simulink model "MPSK_sample_based"  (R2017b)
settings: Solver=FixedStepAuto  StartTime=0.0  StopTime=stopTime  FixedStep=clockTime  RelTol=1e-3
values from neighbouring files (symbols this model uses):
  detectionThreshold = 0.5    [MPSK_frame_based_init.m]    (also in MPSK_sample_based_init.m)
  M = 2^K    (= 4)    [Digital_QAM.m]    (also in MPSK_constellation_decisionRegions.m = 8; MPSK_frame_based_init.m = 2; MPSK_init.m = 2; MPSK_sample_based_init.m = 2)
  phaseOffset = pi    (= 3.14159265359)    [MPSK_frame_based_init.m]    (also in MPSK_init.m = -0.785398163397; MPSK_sample_based_init.m)
  samplesPerSymb = 10    [MPSK_sample_based_init.m]
  sampleTime = 1/sampleRate    (= 0.01)    [MPSK_sample_based_init.m]
undefined symbols (not defined in the file or in its folder): i
libraries: simulink x4, simulink_extras x3, commutil2 x3, dspsigops x2, commfilt2 x2, commchan3 x1, commseqgen3 x1, commsink2 x1, commrflib2 x1
settings Model: Creator=john3  LastModifiedBy=croft

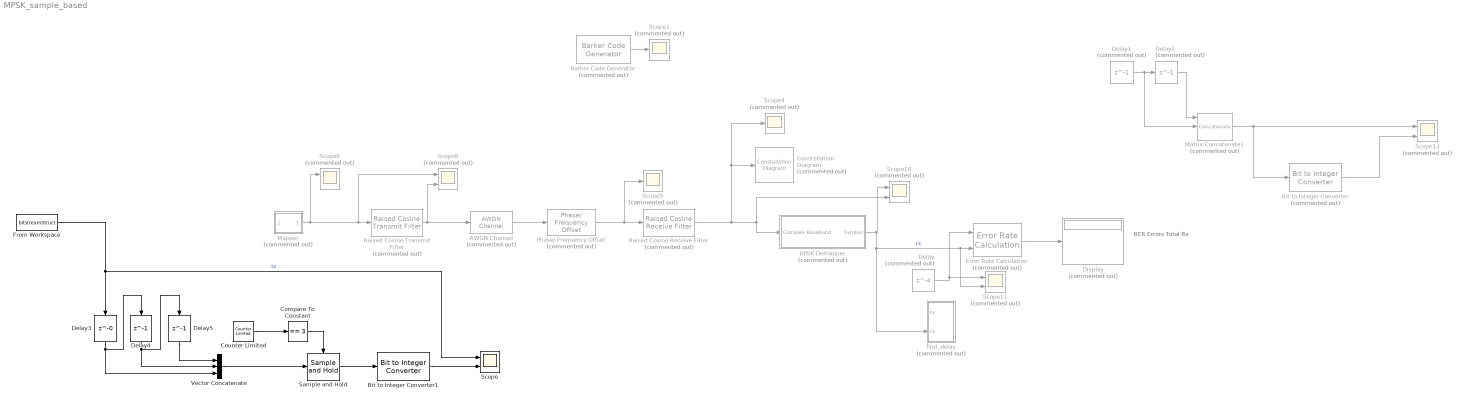
== system MPSK_sample_based ==
  note: BER
      | Errors
      | Total Rx
  AWGN Channel : commchan3/AWGN Channel  Commented=on  InputProcessing=Columns as channels (frame based)  seed=67  noiseMode="Signal to noise ratio  (SNR)"  EbNodB=10  EsNodB=10  SNRdB=30  bitsPerSym=K  Ps=1  Tsym=1  variance=1
  BPSK Demapper : Subsystem  Commented=on
  Barker Code Generator : commseqgen3/Barker Code Generator  Commented=on  Length=7  LengthSimulink=7  SampleTime=1  SamplesPerFrame=1  OutputDataType=double  SimulateUsing=Interpreted execution
      settings: SourceProductName=Communications System Toolbox  SourceProductBaseCode=CM
  Bit to Integer Converter : commutil2/Bit to Integer Converter  Commented=on  nbits=3  bitOrder=MSB first  signedOutputValues=Unsigned  outDtype=Inherit via internal rule  outDtypeSigned=Inherit via internal rule
  Bit to Integer Converter1 : commutil2/Bit to Integer Converter  nbits=3  bitOrder=MSB first  signedOutputValues=Unsigned  outDtype=Inherit via internal rule  outDtypeSigned=Inherit via internal rule
  Compare To Constant : simulink/Logic and Bit Operations/Compare To Constant  relop===  const=3  OutDataTypeStr=boolean
  Constellation Diagram : ConstellationDiagram  Commented=on
  Counter Limited : simulink/Sources/Counter Limited  uplimit=3  tsamp=sampleTime
  Delay : Delay  Commented=on  DelayLength=4
  Delay1 : Delay  Commented=on  DelayLength=1
  Delay2 : Delay  Commented=on  DelayLength=1
  Delay3 : Delay  DelayLength=0
  Delay4 : Delay  DelayLength=1
  Delay5 : Delay  DelayLength=1
  Display : Display  Commented=on
  Error Rate Calculation : commsink2/Error Rate Calculation  Commented=on  N=0  st_delay=0  cp_mode=Entire frame  subframe=[]  PMode=Port  WsName=ErrorVec  RsMode2=off  stop=off  numErr=100  maxBits=1e6
  From Workspace : FromWorkspace  VariableName=bitstreamStruct  SampleTime=sampleTime
  Mapper : Subsystem  Commented=on
  Matrix Concatenate1 : Concatenate  Commented=on  NumInputs=3  ConcatenateDimension=2
  Phase/ Frequency Offset : commrflib2/Phase// Frequency Offset  Commented=on  phaseOffset=phaseOffset*180/pi  freqPort=off  freqOffset=0
      settings: SourceProductName=Communications System Toolbox
  Raised Cosine Receive Filter : commfilt2/Raised Cosine Receive Filter  Commented=on  filtType=Square root  R=1  filtSpan=4  N=samplesPerSymb  downFactor=samplesPerSymb  downOffset=0  filterGain=1  RateOptions=Allow multirate processing  framing=Mute  checkCoeff=off  variableName=rcRxFilt  currentFiltSpan=4  D=(4)/2  inputOffset=0  sampMode=Mute  saveAsFlag=0  rateMode=Downsampling  checkGain=Normalized  launchFVT=on  roundingMode=Floor  overflowMode=off  coeffDataTypeStr=Inherit: Same word length as input  coeffMin=[]  coeffMax=[]  coeffLastDataTypeStr=Inherit: Same word length as input  accumDataTypeStr=Inherit: Same as product output  accumLastDataTypeStr=Inherit: Same as product output  outputDataTypeStr=Inherit: Same as accumulator  outputMin=[]  outputMax=[]  outputLastDataTypeStr=Inherit: Same as accumulator
  Raised Cosine Transmit Filter : commfilt2/Raised Cosine Transmit Filter  Commented=on  filtType=Square root  R=1  filtSpan=4  N=samplesPerSymb  filterGain=1  RateOptions=Allow multirate processing  framing=Mute  checkCoeff=off  variableName=rcTxFilt  checkGain=Normalized  sampMode=Mute  saveAsFlag=0  currentFiltSpan=4  D=(4)/2  launchFVT=on  roundingMode=Floor  overflowMode=off  coeffDataTypeStr=Inherit: Same word length as input  coeffMin=[]  coeffMax=[]  coeffLastDataTypeStr=Inherit: Same word length as input  outputDataTypeStr=Inherit: Same as accumulator  outputMin=[]  outputMax=[]  outputLastDataTypeStr=Inherit: Same as accumulator
  Sample and Hold : dspsigops/Sample and Hold  trig=Rising edge  initCond=0  latchinput=off
  Scope : Scope  NumInputPorts=2
  Scope1 : Scope  Commented=on
  Scope{6,8,10..11,13} (5 alike) : Scope  Commented=on  NumInputPorts=2
  Scope4 : Scope  Commented=on
  Scope9 : Scope  Commented=on
  Vector Concatenate : Concatenate  NumInputs=3
  find_delay : Subsystem  Commented=on
  wires:
  Error Rate Calculation/1 -> Display/1
  Barker Code Generator/1 -> Scope1/1
  AWGN Channel/1 -> Phase/ Frequency Offset/1
  Mapper/1(Out1) -> Scope8/1, Raised Cosine Transmit Filter/1, Scope6/1
  Raised Cosine Transmit Filter/1 -> AWGN Channel/1, Scope8/2
  Phase/ Frequency Offset/1 -> Raised Cosine Receive Filter/1, Scope9/1
  Raised Cosine Receive Filter/1 -> Scope10/2, BPSK Demapper/1(Complex Baseband), Scope4/1, Constellation Diagram/1
  BPSK Demapper/1(Symbol) -> Scope11/2, Error Rate Calculation/2, find_delay/2(rx), Scope10/1  "rx"
  Delay1/1 -> Matrix Concatenate1/2, Delay2/1
  Delay2/1 -> Matrix Concatenate1/1
  Bit to Integer Converter/1 -> Scope13/2
  Matrix Concatenate1/1 -> Scope13/1, Bit to Integer Converter/1
  Delay/1 -> Scope11/1, Error Rate Calculation/1
  From Workspace/1 -> Scope/1, Delay3/1  "tx"
  Delay3/1 -> Vector Concatenate/3, Delay4/1
  Delay4/1 -> Vector Concatenate/2, Delay5/1
  Delay5/1 -> Vector Concatenate/1
  Counter Limited/1 -> Compare To Constant/1
  Compare To Constant/1 -> Sample and Hold/Trigger
  Vector Concatenate/1 -> Sample and Hold/1
  Sample and Hold/1 -> Bit to Integer Converter1/1
  Bit to Integer Converter1/1 -> Scope/2

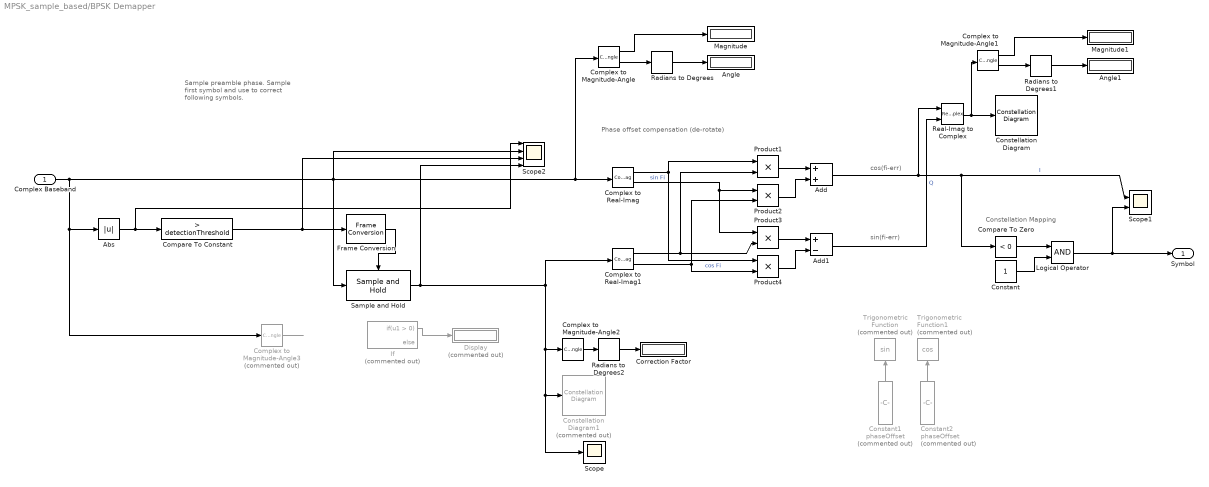
== system MPSK_sample_based/BPSK Demapper ==
  note: cos(fi-err)
  note: Sample preamble phase.
      | Sample first symbol and
      | use to correct following
      | symbols.
  note: Phase offset compensation (de-rotate)
  note: Constellation Mapping
  note: sin(fi-err)
  Complex Baseband : Inport
  Abs : Abs
  Add : Sum
  Add1 : Sum  Inputs=+-
  Angle : Display
  Angle1 : Display
  Compare To Constant : simulink/Logic and Bit Operations/Compare To Constant  relop=>  const=detectionThreshold  OutDataTypeStr=boolean
  Compare To Zero : simulink/Logic and Bit Operations/Compare To Zero  relop=<  OutDataTypeStr=boolean
  Complex to Magnitude-Angle : ComplexToMagnitudeAngle
  Complex to Magnitude-Angle1 : ComplexToMagnitudeAngle
  Complex to Magnitude-Angle2 : ComplexToMagnitudeAngle  Output=Angle
  Complex to Magnitude-Angle3 : ComplexToMagnitudeAngle  Commented=on  Output=Angle
  Complex to Real-Imag : ComplexToRealImag
  Complex to Real-Imag1 : ComplexToRealImag
  Constant : Constant  OutDataTypeStr=boolean
  Constant1 : Constant  Commented=on  Value=phaseOffset
  Constant2 : Constant  Commented=on  Value=phaseOffset
  Constellation Diagram : ConstellationDiagram
  Constellation Diagram1 : ConstellationDiagram  Commented=on
  Correction Factor : Display
  Display : Display  Commented=on
  Frame Conversion : FrameConversion  InheritSamplingMode=off  OutFrame=Sample-based
  If : If  Commented=on
  Logical Operator : Logic  AllPortsSameDT=off  OutDataTypeStr=boolean
  Magnitude : Display
  Magnitude1 : Display
  Product{1..4} (4 alike) : Product
  Radians to Degrees : simulink_extras/Transformations/Radians to Degrees
  Radians to Degrees1 : simulink_extras/Transformations/Radians to Degrees
  Radians to Degrees2 : simulink_extras/Transformations/Radians to Degrees
  Real-Imag to Complex : RealImagToComplex
  Sample and Hold : dspsigops/Sample and Hold  trig=Rising edge  initCond=0  latchinput=off
  Scope : Scope
  Scope1 : Scope  NumInputPorts=2
  Scope2 : Scope  NumInputPorts=4
  Trigonometric Function : Trigonometry  Commented=on
  Trigonometric Function1 : Trigonometry  Commented=on  Operator=cos
  Symbol : Outport
  wires:
  Compare To Zero/1 -> Logical Operator/1
  Complex Baseband/1 -> Sample and Hold/1, Scope2/2, Complex to Magnitude-Angle/1, Complex to Real-Imag/1, Complex to Magnitude-Angle3/1, Abs/1
  Constant/1 -> Logical Operator/2
  Constant1/1 -> Trigonometric Function/1
  Constant2/1 -> Trigonometric Function1/1
  Real-Imag to Complex/1 -> Complex to Magnitude-Angle1/1, Constellation Diagram/1
  Product1/1 -> Add/1
  Product2/1 -> Add/2
  Product3/1 -> Add1/1
  Product4/1 -> Add1/2
  Add/1 -> Compare To Zero/1, Scope1/1, Real-Imag to Complex/1  "I"
  Add1/1 -> Real-Imag to Complex/2  "Q"
  Logical Operator/1 -> Scope1/2, Symbol/1
  Sample and Hold/1 -> Scope2/4, Scope/1, Constellation Diagram1/1, Complex to Magnitude-Angle2/1, Complex to Real-Imag1/1
  Complex to Magnitude-Angle/1 -> Magnitude/1
  Complex to Magnitude-Angle/2 -> Radians to Degrees/1
  Radians to Degrees/1 -> Angle/1
  Radians to Degrees1/1 -> Angle1/1
  Complex to Magnitude-Angle1/2 -> Radians to Degrees1/1
  Complex to Magnitude-Angle1/1 -> Magnitude1/1
  Complex to Magnitude-Angle2/1 -> Radians to Degrees2/1
  Radians to Degrees2/1 -> Correction Factor/1
  Complex to Real-Imag/1 -> Product4/1, Product1/1  "cos Fi"
  Complex to Real-Imag1/1 -> Product3/2, Product1/2
  Complex to Real-Imag/2 -> Product3/1, Product2/1  "sin Fi"
  Complex to Real-Imag1/2 -> Product4/2, Product2/2
  If/1 -> Display/1
  Complex to Magnitude-Angle3/1 -> ?
  ? -> If/1
  Abs/1 -> Scope2/1, Compare To Constant/1
  Compare To Constant/1 -> Scope2/3, Frame Conversion/1
  Frame Conversion/1 -> Sample and Hold/Trigger

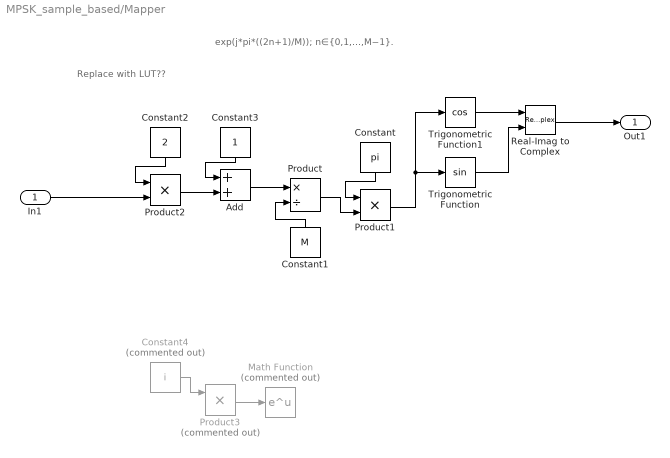
== system MPSK_sample_based/Mapper ==
  note: Replace with LUT??
  note: exp(j*pi*((2n+1)/M)); n∈{0,1,…,M−1}.
  In1 : Inport
  Add : Sum
  Constant : Constant  Value=pi
  Constant1 : Constant  Value=M
  Constant2 : Constant  Value=2
  Constant3 : Constant
  Constant4 : Constant  Commented=on  Value=i
  Math Function : Math  Commented=on  SaturateOnIntegerOverflow=on
  Product : Product  Inputs=*/
  Product1 : Product
  Product2 : Product
  Product3 : Product  Commented=on
  Real-Imag to Complex : RealImagToComplex
  Trigonometric Function : Trigonometry  ApproximationMethod=CORDIC
  Trigonometric Function1 : Trigonometry  Operator=cos  ApproximationMethod=CORDIC
  Out1 : Outport
  wires:
  Real-Imag to Complex/1 -> Out1/1
  Constant2/1 -> Product2/1
  In1/1 -> Product2/2
  Product1/1 -> Trigonometric Function1/1, Trigonometric Function/1
  Trigonometric Function1/1 -> Real-Imag to Complex/1
  Add/1 -> Product/1
  Product/1 -> Product1/2
  Constant3/1 -> Add/1
  Constant1/1 -> Product/2
  Trigonometric Function/1 -> Real-Imag to Complex/2
  Product2/1 -> Add/2
  Constant/1 -> Product1/1
  Constant4/1 -> Product3/1
  Product3/1 -> Math Function/1

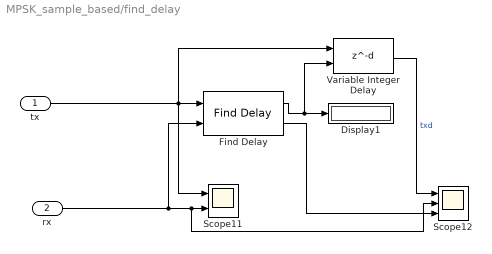
== system MPSK_sample_based/find_delay ==
  tx : Inport
  rx : Inport  Port=2
  Display1 : Display
  Find Delay : commutil2/Find Delay  corrLength=100  chgSigOP=on  stopUpdate=off  numConstDelay=3
      settings: SourceProductName=Communications System Toolbox  SourceProductBaseCode=CM
  Scope11 : Scope  NumInputPorts=2
  Scope12 : Scope  NumInputPorts=3
  Variable Integer Delay : Delay  DelayLengthSource=Input port  SampleTime=sampleTime
      settings: InputPortMap=u0,p1
  wires:
  tx/1 -> Variable Integer Delay/1, Scope11/1, Find Delay/1
  rx/1 -> Find Delay/2, Scope12/2, Scope11/2
  Find Delay/2 -> Scope12/3
  Variable Integer Delay/1 -> Scope12/1  "txd"
  Find Delay/1 -> Variable Integer Delay/2, Display1/1
